simulink library "Delft_Tyre_dtlib"  (Simulink 6.4)
libraries: Delft_Tyre_sm1glib x2
settings Model: Creator=kozlowskimk  LastModifiedBy=hofstadrhmtvd

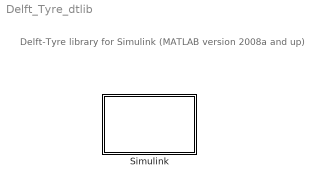
== system Delft_Tyre_dtlib ==
  note: Delft-Tyre library for Simulink
      | (MATLAB version 2008a and up)
  Simulink : Subsystem

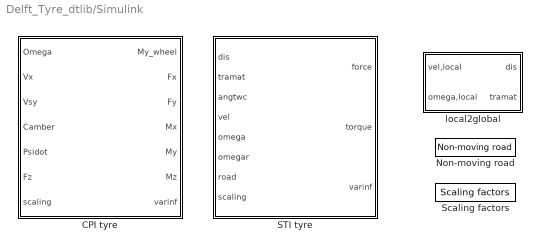
== system Delft_Tyre_dtlib/Simulink ==
  CPI tyre : Subsystem  Tag=CPI tyre  mask(CPI_tyre){idtyre=1, tpfname=, side_mode=(1xxx) left, dyn_mode=(xx0x) steady-state, mf_mode=(xxx0) none, use_mode=1e8, disp_debug=off}
      mask prompts: idtyre "Tyre ID [integer]"; tpfname "Tyre property file [string]"; side_mode "Tyre side            :"; dyn_mode "Dynamics           :"; mf_mode "Slip forces          :"; use_mode "Optional: use mode (overrides pop-up) [integer]"; disp_debug "Display debug messages"
      mask help:
      | Tyre model using the contact point interface (CPI). Inputs to the tyre model are the sliding velocities at the tyre-road contact point.
      |
      | Tyre model version: MF-Tyre/MF-Swift 6.2
      | © 1996-2013 TNO, Helmond, The Netherlands
      mask init:
      | if (abs(use_mode) > 4535 )
      |   iswtch=1000*side_mode+10*(dyn_mode-1)+(mf_mode-1);
      |   if (disp_debug) disp(['Delft-Tyre ' num2str(idtyre) ' -> use_mode=' num2str(iswtch) ]); end
      | else
      |   iswtch=use_mode;
      | end
      | 
      | 
      | if ~exist(tpfname)
      |     error('Tyre property file does not exist') 
      | end
      mask Help: eval('DTOpenHelp(504)')
      mask StyleString: edit,edit,popup((1xxx) left|(2xxx) right|(3xxx) symmetric),popup((xx0x) steady-state|(xx1x) relaxation behaviour|(xx2x) relaxation behaviour - non-linear),popup((xxx0) none|(xxx1) longitudinal|(xxx2) lateral|(xxx3) uncombined|(xxx4) combined|(xxx5) combined+turnslip),edit,checkbox
      mask CallbackString:
      | ||promtstr = get_param(gcb,'MaskPromptString');
      | index = find(double(promtstr)==124);
      | maskval = get_param(gcb,'MaskValues');
      | new_mode = [maskval{3}(2) '0' maskval{4}(4) maskval{5}(5)];
      | newpromtstr = [promtstr(1:index(5)) ['Optional: use mode (overrides pop-up) [current selection: ' new_mode ']'] promtstr(index(6):end)];
      | set_param(gcb,'MaskPromptString',newpromtstr);|promtstr = get_param(gcb,'MaskPromptString');
      | index = find(double(promtstr)==124);
      | maskval = get_param(gcb,'MaskValues');
      | new_mode = [maskval{3}(2) '0' maskval{4}(4) maskval{5}(5)];
      | newpromtstr = [promtstr(1:index(5)) ['Optional: use mode (overrides pop-up) [current selection: ' new_mode ']'] promtstr(index(6):end)];
      | set_param(gcb,'MaskPromptString',newpromtstr);|promtstr = get_param(gcb,'MaskPromptString');
      | index = find(double(promtstr)==124);
      | maskval = get_param(gcb,'MaskValues');
      | new_mode = [maskval{3}(2) '0' maskval{4}(4) maskval{5}(5)];
      | newpromtstr = [promtstr(1:index(5)) ['Optional: use mode (overrides pop-up) [current selection: ' new_mode ']'] promtstr(index(6):end)];
      | set_param(gcb,'MaskPromptString',newpromtstr);||
      mask Display:
      | text(0.3*160,0.7*178,'TNO Delft-Tyre')
      | plot(89.*[0.8828 0.8769 0.8597 0.7299 0.7043 0.6745 0.6443 0.6195 0.5884 0.5712 0.5653 0.5573 0.5346 0.4985 0.4515 0.3965 0.3373 ]+160/2-0.43*89,89.*[0.3654 0.3482 0.3335 0.2583 0.2486 0.2453 0.2486 0.2583 0.2764 0.2911 0.3083 0.2449 0.1945 0.1609 0.1462 0.1520 0.1768 ]+0.3*89)
      | plot(89.*[0.3255 0.3889 0.3965 0.4112 0.4313 0.3767 ]+160/2-0.43*89,89.*[0.1491 0.1222 0.1520 0.1777 0.1949 0.2184 ]+0.3*89)
      | plot(89.*[0.3553 0.4112 0.4633 0.4826 0.5464 ]+160/2-0.43*89,89.*[0.2012 0.1777 0.1722 0.1898 0.2268 ]+0.3*89)
      | plot(89.*[0.5426 0.5262 0.4826 0.4313 0.5603 0.5603 0.5065 ]+160/2-0.43*89,89.*[0.2184 0.2037 0.1898 0.1949 0.2692 0.2701 0.2932 ]+0.3*89)
      | plot(89.*[0.5279 0.5460 0.4868 ]+160/2-0.43*89,89.*[0.3007 0.2969 0.3402 ]+0.3*89)
      | plot(89.*[0.5279 0.5624 ]+160/2-0.43*89,89.*[0.3007 0.2856 ]+0.3*89)
      | plot(89.*[0.5628 0.5460 ]+160/2-0.43*89,89.*[0.2898 0.2969 ]+0.3*89)
      | plot(89.*[0.5712 0.5628 0.5573 ]+160/2-0.43*89,89.*[0.2911 0.2222 0.2449 ]+0.3*89)
      | plot(89.*[0.5586 0.5422 0.5082 0.4633 0.4515 0.4481 0.3889 0.3902 0.4544 0.5099 0.5523 0.5792 0.5884 ]+160/2-0.43*89,89.*[0.2541 0.2180 0.1861 0.1722 0.1462 0.1163 0.1222 0.0928 0.0865 0.1033 0.1428 0.2016 0.2764 ]+0.3*89)
      | plot(89.*[0.6195 0.6090 0.5792 0.5628 0.5380 0.5346 0.5422 ]+160/2-0.43*89,89.*[0.2583 0.1751 0.2016 0.2222 0.1680 0.1945 0.2180 ]+0.3*89)
      | plot(89.*[0.5262 0.5082 0.4985 0.4994 0.5380 0.5523 0.5792 0.6090 0.6333 0.6443 ]+160/2-0.43*89,89.*[0.2037 0.1861 0.1609 0.1319 0.1680 0.1428 0.1092 0.1751 0.1596 0.2486 ]+0.3*89)
      | plot(89.*[0.6745 0.6627 0.6333 0.6018 0.5792 0.5317 0.5099 0.4994 0.4481 0.4544 0.4700 0.5317 0.5510 0.6018 0.6291 0.6627 0.6926 0.7043 ]+160/2-0.43*89,89.*[0.2453 0.1508 0.1596 0.0890 0.1092 0.0655 0.1033 0.1319 0.1163 0.0865 0.0462 0.0655 0.0416 0.0890 0.0764 0.1508 0.1508 0.2486 ]+0.3*89)
      | plot(89.*[0.7299 0.7178 0.6926 0.6577 0.6291 0.5758 0.5510 0.4851 0.4700 0.3986 0.3213 0.2440 0.1718 0.1100 0.0626 ]+160/2-0.43*89,89.*[0.2583 0.1596 0.1508 0.0739 0.0764 0.0269 0.0416 0.0210 0.0462 0.0533 0.0861 0.1424 0.2184 0.3087 0.4074 ]+0.3*89)
      | plot(89.*[0.0487 0.0995 0.1100 0.1323 0.1516 0.1760 0.1399 ]+160/2-0.43*89,89.*[0.4082 0.3028 0.3087 0.3213 0.3326 0.3469 0.4221 ]+0.3*89)
      | plot(89.*[0.1126 0.1516 0.2024 0.2234 0.2474 0.2709 0.4011 0.4200 0.4322 0.3847 0.3486 0.3255 ]+160/2-0.43*89,89.*[0.4141 0.3326 0.2579 0.2776 0.2969 0.3121 0.3872 0.3965 0.3982 0.4670 0.5426 0.6191 ]+0.3*89)
      | plot(89.*[0.3486 0.3410 0.3755 0.3847 ]+160/2-0.43*89,89.*[0.5426 0.5330 0.4616 0.4670 ]+0.3*89)
      | plot(89.*[0.3755 0.3570 0.3234 ]+160/2-0.43*89,89.*[0.4616 0.4511 0.5212 ]+0.3*89)
      | plot(89.*[0.3570 0.2272 0.1936 ]+160/2-0.43*89,89.*[0.4511 0.3759 0.4460 ]+0.3*89)
      | plot(89.*[0.1684 0.2029 0.2272 0.2709 0.3217 0.4519 0.4721 0.4868 0.4322 ]+160/2-0.43*89,89.*[0.4334 0.3625 0.3759 0.3121 0.2583 0.3331 0.3415 0.3402 0.3982 ]+0.3*89)
      | plot(89.*[0.4200 0.3755 ]+160/2-0.43*89,89.*[0.3965 0.4616 ]+0.3*89)
      | plot(89.*[0.3570 0.4011 0.4519 0.5065 0.5279 0.4721 0.4200 ]+160/2-0.43*89,89.*[0.4511 0.3872 0.3331 0.2932 0.3007 0.3415 0.3965 ]+0.3*89)
      | plot(89.*[0.5065 0.3767 0.3217 0.2995 0.2474 0.2029 0.1760 0.2234 0.2785 0.2995 0.3553 0.3767 ]+160/2-0.43*89,89.*[0.2932 0.2184 0.2583 0.2419 0.2969 0.3625 0.3469 0.2776 0.2197 0.2419 0.2012 0.2184 ]+0.3*89)
      | plot(89.*[0.3553 0.3373 0.2785 0.2617 0.2024 0.1873 0.1323 0.0899 0.0630 0.0542 0.0231 0.0059 0.0000 0.0113 0.0168 0.0332 0.0630 0.0878 0.1172 0.1470 0.1722 0.3024 0.3192 0.3255 0.3179 0.3121 0.2948 0.1651 0.1394 0.1470 0.1172 0.0878 0.0630 0.0332 0.0168 0.0113 0.0000 ]+160/2-0.43*89,89.*[0.2012 0.1768 0.2197 0.1957 0.2579 0.2402 0.3213 0.4099 0.4994 0.5846 0.6027 0.6174 0.6346 0.5271 0.5157 0.5078 0.4994 0.4964 0.4990 0.5061 0.5174 0.5922 0.6056 0.6191 0.6917 0.6745 0.6598 0.5846 0.5745 0.6350 0.6350 0.6434 0.6594 0.6858 0.7064 0.7291 0.6346 ]+0.3*89)
      | plot(89.*[0.0059 0.0168 ]+160/2-0.43*89,89.*[0.6174 0.7064 ]+0.3*89)
      | plot(89.*[0.0113 0.0454 0.0529 0.0181 0.0113 ]+160/2-0.43*89,89.*[0.7291 0.8034 0.8270 0.7497 0.7291 ]+0.3*89)
      | plot(89.*[0.0168 0.0487 0.0454 ]+160/2-0.43*89,89.*[0.7064 0.7770 0.8034 ]+0.3*89)
      | plot(89.*[0.0487 0.0626 0.0899 0.0630 0.0542 0.0794 0.0878 0.1126 0.0899 ]+160/2-0.43*89,89.*[0.7770 0.7518 0.7182 0.6594 0.5846 0.5745 0.6434 0.6976 0.7182 ]+0.3*89)
      | plot(89.*[0.1126 0.1399 0.1684 0.1936 0.2570 ]+160/2-0.43*89,89.*[0.6976 0.6854 0.6829 0.6905 0.7274 ]+0.3*89)
      | plot(89.*[0.3011 0.1722 0.1936 ]+160/2-0.43*89,89.*[0.7182 0.6438 0.6905 ]+0.3*89)
      | plot(89.*[0.1684 0.1470 0.1722 0.1651 0.1722 0.1936 0.3234 0.3410 0.3192 0.3121 0.3163 ]+160/2-0.43*89,89.*[0.6829 0.6350 0.6438 0.5846 0.5174 0.4460 0.5212 0.5330 0.6056 0.6745 0.7119 ]+0.3*89)
      | plot(89.*[0.3200 0.3179 ]+160/2-0.43*89,89.*[0.7102 0.6917 ]+0.3*89)
      | plot(89.*[0.3020 0.2948 0.3024 0.3234 ]+160/2-0.43*89,89.*[0.7178 0.6598 0.5922 0.5212 ]+0.3*89)
      | plot(89.*[0.1470 0.1394 0.1096 0.1172 0.1399 0.1760 0.1516 0.1323 0.1100 0.0995 0.0987 0.1688 0.1806 0.1999 0.3297 0.2566 0.1264 0.0701 0.0529 0.1084 0.1264 0.1999 ]+160/2-0.43*89,89.*[0.5061 0.5745 0.5716 0.6350 0.6854 0.7190 0.7341 0.7577 0.7959 0.8240 0.8530 0.8748 0.9005 0.9185 0.9933 0.9706 0.8958 0.8438 0.8270 0.8782 0.8958 0.9185 ]+0.3*89)
      | plot(89.*[0.1806 0.1084 0.0987 0.0454 ]+160/2-0.43*89,89.*[0.9005 0.8782 0.8530 0.8034 ]+0.3*89)
      | plot(89.*[0.0487 0.0995 0.1655 0.1688 ]+160/2-0.43*89,89.*[0.7770 0.8240 0.8446 0.8748 ]+0.3*89)
      | plot(89.*[0.1655 0.1718 0.1873 0.2024 0.2234 0.2474 0.2029 0.1760 0.2234 ]+160/2-0.43*89,89.*[0.8446 0.8148 0.7745 0.7497 0.7333 0.7283 0.7144 0.7190 0.7333 ]+0.3*89)
      | plot(89.*[0.2272 0.2478 ]+160/2-0.43*89,89.*[0.7215 0.7278 ]+0.3*89)
      | plot(89.*[0.2272 0.2029 0.1684 ]+160/2-0.43*89,89.*[0.7215 0.7144 0.6829 ]+0.3*89)
      | plot(89.*[0.1936 0.2272 ]+160/2-0.43*89,89.*[0.6905 0.7215 ]+0.3*89)
      | plot(89.*[0.2024 0.1516 0.1126 ]+160/2-0.43*89,89.*[0.7497 0.7341 0.6976 ]+0.3*89)
      | plot(89.*[0.0899 0.1323 0.1873 0.2520 0.2440 0.2428 0.2499 0.2650 0.2852 0.4150 0.4372 0.3528 0.3297 0.4150 0.5065 0.5279 0.5460 0.4586 0.4372 0.5279 ]+160/2-0.43*89,89.*[0.7182 0.7577 0.7745 0.7686 0.8076 0.8370 0.8669 0.8925 0.9097 0.9849 0.9920 1.0000 0.9933 0.9849 0.9458 0.9534 0.9500 0.9870 0.9920 0.9534 ]+0.3*89)
      | plot(89.*[0.5065 0.3767 0.2852 0.1999 ]+160/2-0.43*89,89.*[0.9458 0.8711 0.9097 0.9185 ]+0.3*89)
      | plot(89.*[0.1806 0.2650 0.3553 0.3767 ]+160/2-0.43*89,89.*[0.9005 0.8925 0.8538 0.8711 ]+0.3*89)
      | plot(89.*[0.3553 0.3373 0.2499 0.1688 ]+160/2-0.43*89,89.*[0.8538 0.8295 0.8669 0.8748 ]+0.3*89)
      | plot(89.*[0.1655 0.2428 0.3255 0.3373 ]+160/2-0.43*89,89.*[0.8446 0.8370 0.8018 0.8295 ]+0.3*89)
      | plot(89.*[0.3255 0.3213 0.3213 0.3255 0.3373 0.2785 0.2617 0.3255 ]+160/2-0.43*89,89.*[0.8018 0.7749 0.7388 0.7165 0.7031 0.7278 0.7438 0.7165 ]+0.3*89)
      | plot(89.*[0.3213 0.2520 0.2617 0.2024 ]+160/2-0.43*89,89.*[0.7388 0.7686 0.7438 0.7497 ]+0.3*89)
      | plot(89.*[0.2234 0.2785 ]+160/2-0.43*89,89.*[0.7333 0.7278 ]+0.3*89)
      | plot(89.*[0.2869 0.2474 ]+160/2-0.43*89,89.*[0.7241 0.7283 ]+0.3*89)
      | plot(89.*[0.2440 0.3213 0.3986 0.4078 0.4246 0.4456 0.4683 0.5981 0.6182 0.6329 0.5460 ]+160/2-0.43*89,89.*[0.8076 0.7749 0.7186 0.7417 0.7661 0.7879 0.8043 0.8790 0.8874 0.8862 0.9500 ]+0.3*89)
      | plot(89.*[0.5279 0.6182 0.7022 0.7140 0.6329 ]+160/2-0.43*89,89.*[0.9534 0.8874 0.7984 0.8001 0.8862 ]+0.3*89)
      | plot(89.*[0.5981 0.5065 ]+160/2-0.43*89,89.*[0.8790 0.9458 ]+0.3*89)
      | plot(89.*[0.5981 0.6829 0.7022 ]+160/2-0.43*89,89.*[0.8790 0.7892 0.7984 ]+0.3*89)
      | plot(89.*[0.6829 0.5535 0.4683 0.3767 ]+160/2-0.43*89,89.*[0.7892 0.7144 0.8043 0.8711 ]+0.3*89)
      | plot(89.*[0.3553 0.4456 0.5300 0.5535 ]+160/2-0.43*89,89.*[0.8538 0.7879 0.6989 0.7144 ]+0.3*89)
      | plot(89.*[0.5300 0.5061 0.4246 0.3373 ]+160/2-0.43*89,89.*[0.6989 0.6800 0.7661 0.8295 ]+0.3*89)
      | plot(89.*[0.3255 0.4078 0.4851 0.5061 ]+160/2-0.43*89,89.*[0.8018 0.7417 0.6602 0.6800 ]+0.3*89)
      | plot(89.*[0.4851 0.4700 0.3986 0.3902 0.3889 0.4481 0.4544 0.4700 ]+160/2-0.43*89,89.*[0.6602 0.6426 0.7186 0.6884 0.6703 0.6077 0.6203 0.6426 ]+0.3*89)
      | plot(89.*[0.4851 0.5510 0.5758 0.6027 0.6262 0.7560 0.7745 0.7841 0.7140 ]+160/2-0.43*89,89.*[0.6602 0.5632 0.5779 0.5930 0.6069 0.6816 0.6926 0.6980 0.8001 ]+0.3*89)
      | plot(89.*[0.7022 0.7745 ]+160/2-0.43*89,89.*[0.7984 0.6926 ]+0.3*89)
      | plot(89.*[0.7841 0.8375 0.8303 0.7745 ]+160/2-0.43*89,89.*[0.6980 0.5863 0.5766 0.6926 ]+0.3*89)
      | plot(89.*[0.7560 0.6829 ]+160/2-0.43*89,89.*[0.6816 0.7892 ]+0.3*89)
      | plot(89.*[0.7560 0.8123 0.8303 ]+160/2-0.43*89,89.*[0.6816 0.5649 0.5766 ]+0.3*89)
      | plot(89.*[0.8123 0.6825 0.6262 0.5535 ]+160/2-0.43*89,89.*[0.5649 0.4901 0.6069 0.7144 ]+0.3*89)
      | plot(89.*[0.5300 0.6027 0.6577 0.6825 ]+160/2-0.43*89,89.*[0.6989 0.5930 0.4775 0.4901 ]+0.3*89)
      | plot(89.*[0.6577 0.6291 0.5758 0.5061 ]+160/2-0.43*89,89.*[0.4775 0.4658 0.5779 0.6800 ]+0.3*89)
      | plot(89.*[0.4700 0.5317 0.5510 0.6018 0.6291 ]+160/2-0.43*89,89.*[0.6426 0.5523 0.5632 0.4578 0.4658 ]+0.3*89)
      | plot(89.*[0.6018 0.5792 0.5317 0.5099 0.4544 0.3902 0.3213 ]+160/2-0.43*89,89.*[0.4578 0.4536 0.5523 0.5397 0.6203 0.6884 0.7388 ]+0.3*89)
      | plot(89.*[0.3255 0.3889 0.3965 0.4515 0.4481 0.4994 0.5099 0.5523 0.5792 ]+160/2-0.43*89,89.*[0.7165 0.6703 0.6602 0.6018 0.6077 0.5334 0.5397 0.4511 0.4536 ]+0.3*89)
      | plot(89.*[0.6018 0.6333 0.6627 0.6926 0.7178 0.8475 0.8652 0.8711 0.8375 ]+160/2-0.43*89,89.*[0.4578 0.3503 0.3524 0.3599 0.3713 0.4460 0.4595 0.4729 0.5863 ]+0.3*89)
      | plot(89.*[0.8303 0.8652 ]+160/2-0.43*89,89.*[0.5766 0.4595 ]+0.3*89)
      | plot(89.*[0.8711 0.8828 0.8711 0.8652 0.8475 0.7178 0.6825 0.6577 0.6027 0.5758 0.5061 0.4851 0.4078 0.3986 0.3902 0.3213 0.2520 0.1873 0.1718 0.1655 0.0995 0.0987 0.1688 0.1655 0.2428 0.2440 0.2520 0.2617 0.3255 0.3373 ]+160/2-0.43*89,89.*[0.4729 0.3654 0.2713 0.2503 0.2348 0.1596 0.0815 0.0739 0.0223 0.0269 0.0050 0.0210 0.0290 0.0533 0.0928 0.1222 0.1726 0.2402 0.2184 0.2058 0.3028 0.3020 0.1999 0.2058 0.1243 0.1424 0.1726 0.1957 0.1491 0.1768 ]+0.3*89)
      | plot(89.*[0.3255 0.3213 0.3213 0.3255 0.4078 0.4246 0.5061 0.5300 0.6027 0.6262 0.6825 0.8123 0.8475 0.8597 0.8475 0.8123 ]+160/2-0.43*89,89.*[0.1491 0.1222 0.0861 0.0643 0.0290 0.0130 0.0050 0.0000 0.0223 0.0294 0.0815 0.1562 0.2348 0.3335 0.4460 0.5649 ]+0.3*89)
      | plot(89.*[0.8652 0.8769 0.8652 0.8303 0.8123 0.7560 0.6262 0.5535 0.5300 0.4456 0.4246 0.3373 0.3255 0.2428 0.2499 0.3373 ]+160/2-0.43*89,89.*[0.4595 0.3482 0.2503 0.1735 0.1562 0.1046 0.0294 0.0067 0.0000 0.0084 0.0130 0.0504 0.0643 0.1243 0.1138 0.0504 ]+0.3*89)
      | plot(89.*[0.0487 0.0168 0.0059 ]+160/2-0.43*89,89.*[0.4082 0.5157 0.6174 ]+0.3*89)
      | plot(89.*[0.0231 0.0332 0.0626 0.1100 0.1718 0.2440 ]+160/2-0.43*89,89.*[0.6027 0.6858 0.7518 0.7959 0.8148 0.8076 ]+0.3*89)
      | plot(89.*[0.3373 0.3965 ]+160/2-0.43*89,89.*[0.7031 0.6602 ]+0.3*89)
      | plot(89.*[0.4515 0.4985 0.4994 0.5380 0.5523 0.5792 0.6090 0.6333 0.6443 ]+160/2-0.43*89,89.*[0.6018 0.5330 0.5334 0.4519 0.4511 0.3612 0.3532 0.3503 0.2486 ]+0.3*89)
      | plot(89.*[0.6745 0.6627 0.6291 ]+160/2-0.43*89,89.*[0.2453 0.3524 0.4658 ]+0.3*89)
      | plot(89.*[0.6577 0.6926 0.7043 ]+160/2-0.43*89,89.*[0.4775 0.3599 0.2486 ]+0.3*89)
      | plot(89.*[0.7299 0.7178 0.6825 ]+160/2-0.43*89,89.*[0.2583 0.3713 0.4901 ]+0.3*89)
      | plot(89.*[0.5792 0.6090 0.6195 ]+160/2-0.43*89,89.*[0.4536 0.3532 0.2583 ]+0.3*89)
      | plot(89.*[0.5884 0.5792 0.5628 0.5380 0.5346 0.5573 0.5628 0.5712 ]+160/2-0.43*89,89.*[0.2764 0.3612 0.3692 0.4519 0.4578 0.3809 0.3692 0.2911 ]+0.3*89)
      | plot(89.*[0.5653 0.5573 ]+160/2-0.43*89,89.*[0.3083 0.3809 ]+0.3*89)
      | plot(89.*[0.5346 0.4985 ]+160/2-0.43*89,89.*[0.4578 0.5330 ]+0.3*89)
      | plot(89.*[0.1470 0.1684 0.1936 ]+160/2-0.43*89,89.*[0.5061 0.4334 0.4460 ]+0.3*89)
      | plot(89.*[0.1684 0.1399 0.1172 0.1096 0.0794 0.0878 0.1126 0.1399 ]+160/2-0.43*89,89.*[0.4334 0.4221 0.4990 0.5716 0.5745 0.4964 0.4141 0.4221 ]+0.3*89)
      | plot(89.*[0.1126 0.0899 0.0626 0.0332 0.0231 ]+160/2-0.43*89,89.*[0.4141 0.4099 0.4074 0.5078 0.6027 ]+0.3*89)
      | plot(89.*[0.0113 0.0454 0.0487 0.0626 ]+160/2-0.43*89,89.*[0.5271 0.4137 0.4082 0.4074 ]+0.3*89)
      | plot(89.*[0.0454 0.0987 ]+160/2-0.43*89,89.*[0.4137 0.3020 ]+0.3*89)
  Non-moving road : Delft_Tyre_sm1glib/SimMechanics 1G/Non-moving road  Tag=Non-moving road  SystemSampleTime=-1  dummy=off
  STI tyre : Subsystem  Tag=STI tyre  mask(STI_tyre){idtyre=1, tpfname=, rdfname='', side_mode=(1xxx) left, cnt_mode=(x1xx) smooth road, dyn_mode=(xx0x) steady-state, mf_mode=(xxx0) none, use_mode=1e8, disp_debug=off}
      mask prompts: idtyre "Tyre ID [integer]"; tpfname "Tyre properties [string or struct]"; rdfname "Road data file (may be empty) [string]"; side_mode "Tyre side            :"; cnt_mode "Contact method :"; dyn_mode "Dynamics           :"; mf_mode "Slip forces          :"; use_mode "Optional: use mode (overrides pop-up) [integer]"; disp_debug "Display debug messages"
      mask help:
      | Tyre model using the standard tyre interface (STI), as developed by the TYDEX workgroup. Inputs to the tyre model are the motions at the wheel centre. The outputs force and torque should also be applied to the wheel centre.
      |
      | Tyre model version: MF-Tyre/MF-Swift 6.2
      | © 1996-2013 TNO, Helmond, The Netherlands
      mask init:
      | idroad=1;
      | if (abs(use_mode) > 4535 )
      |   iswtch=1000*side_mode+100*cnt_mode+10*(dyn_mode-1)+(mf_mode-1);
      |   if (disp_debug) disp(['Delft-Tyre ' num2str(idtyre) ' -> use_mode=' num2str(iswtch) ]); end
      | else
      |   iswtch=use_mode;
      | end
      | 
      | % switch between tpf file or struct
      | if ischar(tpfname)
      |     typarr=zeros(300,1);
      |     tpfname_dummy=tpfname;
      | elseif isstruct(tpfname)
      |     typarr=tno_tpf_struct2array(tpfname,idtyre);
      |     tpfname_dummy='';
      | else
      |     typarr=zeros(300,1);
      |     tpfname_dummy='';
      |     error(['Mask parameter ''Tyre property file'' should be supplied as string or structure for tyre ' num2str(idtyre)])
      | end
      mask Help: eval('DTOpenHelp(505)')
      mask StyleString: edit,edit,edit,popup((1xxx) left|(2xxx) right|(3xxx) symmetric),popup((x1xx) smooth road|(x2xx) smooth road (motorcycle: circular cross section)|(x3xx) moving road|(x4xx) 2D short wavelength road contact|(x5xx) 3D short wavelength road contact),popup((xx0x) steady-state|(xx1x) relaxation behaviour|(xx2x) relaxation behaviour - non-linear|(xx3x) rigid ring|(xx4x) rigid ring + initial statics),popup((xxx0) none|(xxx1) longitudinal|(xxx2) lateral|(xxx3) uncombined|(xxx4) combined|(xxx5) combined+turnslip),edit,checkbox
      mask CallbackString:
      | |||promtstr = get_param(gcb,'MaskPromptString');
      | index = find(double(promtstr)==124);
      | maskval = get_param(gcb,'MaskValues');
      | new_mode = [maskval{4}(2) maskval{5}(3) maskval{6}(4) maskval{7}(5)];
      | newpromtstr = [promtstr(1:index(7)) ['Optional: use mode (overrides pop-up) [current selection: ' new_mode ']'] promtstr(index(8):end)];
      | set_param(gcb,'MaskPromptString',newpromtstr);|promtstr = get_param(gcb,'MaskPromptString');
      | index = find(double(promtstr)==124);
      | maskval = get_param(gcb,'MaskValues');
      | new_mode = [maskval{4}(2) maskval{5}(3) maskval{6}(4) maskval{7}(5)];
      | newpromtstr = [promtstr(1:index(7)) ['Optional: use mode (overrides pop-up) [current selection: ' new_mode ']'] promtstr(index(8):end)];
      | set_param(gcb,'MaskPromptString',newpromtstr);|promtstr = get_param(gcb,'MaskPromptString');
      | index = find(double(promtstr)==124);
      | maskval = get_param(gcb,'MaskValues');
      | new_mode = [maskval{4}(2) maskval{5}(3) maskval{6}(4) maskval{7}(5)];
      | newpromtstr = [promtstr(1:index(7)) ['Optional: use mode (overrides pop-up) [current selection: ' new_mode ']'] promtstr(index(8):end)];
      | set_param(gcb,'MaskPromptString',newpromtstr);|promtstr = get_param(gcb,'MaskPromptString');
      | index = find(double(promtstr)==124);
      | maskval = get_param(gcb,'MaskValues');
      | new_mode = [maskval{4}(2) maskval{5}(3) maskval{6}(4) maskval{7}(5)];
      | newpromtstr = [promtstr(1:index(7)) ['Optional: use mode (overrides pop-up) [current selection: ' new_mode ']'] promtstr(index(8):end)];
      | set_param(gcb,'MaskPromptString',newpromtstr);||
      mask Display:
      | text(0.3*160,0.7*178,'TNO Delft-Tyre')
      | plot(89.*[0.8828 0.8769 0.8597 0.7299 0.7043 0.6745 0.6443 0.6195 0.5884 0.5712 0.5653 0.5573 0.5346 0.4985 0.4515 0.3965 0.3373 ]+160/2-0.43*89,89.*[0.3654 0.3482 0.3335 0.2583 0.2486 0.2453 0.2486 0.2583 0.2764 0.2911 0.3083 0.2449 0.1945 0.1609 0.1462 0.1520 0.1768 ]+0.3*89)
      | plot(89.*[0.3255 0.3889 0.3965 0.4112 0.4313 0.3767 ]+160/2-0.43*89,89.*[0.1491 0.1222 0.1520 0.1777 0.1949 0.2184 ]+0.3*89)
      | plot(89.*[0.3553 0.4112 0.4633 0.4826 0.5464 ]+160/2-0.43*89,89.*[0.2012 0.1777 0.1722 0.1898 0.2268 ]+0.3*89)
      | plot(89.*[0.5426 0.5262 0.4826 0.4313 0.5603 0.5603 0.5065 ]+160/2-0.43*89,89.*[0.2184 0.2037 0.1898 0.1949 0.2692 0.2701 0.2932 ]+0.3*89)
      | plot(89.*[0.5279 0.5460 0.4868 ]+160/2-0.43*89,89.*[0.3007 0.2969 0.3402 ]+0.3*89)
      | plot(89.*[0.5279 0.5624 ]+160/2-0.43*89,89.*[0.3007 0.2856 ]+0.3*89)
      | plot(89.*[0.5628 0.5460 ]+160/2-0.43*89,89.*[0.2898 0.2969 ]+0.3*89)
      | plot(89.*[0.5712 0.5628 0.5573 ]+160/2-0.43*89,89.*[0.2911 0.2222 0.2449 ]+0.3*89)
      | plot(89.*[0.5586 0.5422 0.5082 0.4633 0.4515 0.4481 0.3889 0.3902 0.4544 0.5099 0.5523 0.5792 0.5884 ]+160/2-0.43*89,89.*[0.2541 0.2180 0.1861 0.1722 0.1462 0.1163 0.1222 0.0928 0.0865 0.1033 0.1428 0.2016 0.2764 ]+0.3*89)
      | plot(89.*[0.6195 0.6090 0.5792 0.5628 0.5380 0.5346 0.5422 ]+160/2-0.43*89,89.*[0.2583 0.1751 0.2016 0.2222 0.1680 0.1945 0.2180 ]+0.3*89)
      | plot(89.*[0.5262 0.5082 0.4985 0.4994 0.5380 0.5523 0.5792 0.6090 0.6333 0.6443 ]+160/2-0.43*89,89.*[0.2037 0.1861 0.1609 0.1319 0.1680 0.1428 0.1092 0.1751 0.1596 0.2486 ]+0.3*89)
      | plot(89.*[0.6745 0.6627 0.6333 0.6018 0.5792 0.5317 0.5099 0.4994 0.4481 0.4544 0.4700 0.5317 0.5510 0.6018 0.6291 0.6627 0.6926 0.7043 ]+160/2-0.43*89,89.*[0.2453 0.1508 0.1596 0.0890 0.1092 0.0655 0.1033 0.1319 0.1163 0.0865 0.0462 0.0655 0.0416 0.0890 0.0764 0.1508 0.1508 0.2486 ]+0.3*89)
      | plot(89.*[0.7299 0.7178 0.6926 0.6577 0.6291 0.5758 0.5510 0.4851 0.4700 0.3986 0.3213 0.2440 0.1718 0.1100 0.0626 ]+160/2-0.43*89,89.*[0.2583 0.1596 0.1508 0.0739 0.0764 0.0269 0.0416 0.0210 0.0462 0.0533 0.0861 0.1424 0.2184 0.3087 0.4074 ]+0.3*89)
      | plot(89.*[0.0487 0.0995 0.1100 0.1323 0.1516 0.1760 0.1399 ]+160/2-0.43*89,89.*[0.4082 0.3028 0.3087 0.3213 0.3326 0.3469 0.4221 ]+0.3*89)
      | plot(89.*[0.1126 0.1516 0.2024 0.2234 0.2474 0.2709 0.4011 0.4200 0.4322 0.3847 0.3486 0.3255 ]+160/2-0.43*89,89.*[0.4141 0.3326 0.2579 0.2776 0.2969 0.3121 0.3872 0.3965 0.3982 0.4670 0.5426 0.6191 ]+0.3*89)
      | plot(89.*[0.3486 0.3410 0.3755 0.3847 ]+160/2-0.43*89,89.*[0.5426 0.5330 0.4616 0.4670 ]+0.3*89)
      | plot(89.*[0.3755 0.3570 0.3234 ]+160/2-0.43*89,89.*[0.4616 0.4511 0.5212 ]+0.3*89)
      | plot(89.*[0.3570 0.2272 0.1936 ]+160/2-0.43*89,89.*[0.4511 0.3759 0.4460 ]+0.3*89)
      | plot(89.*[0.1684 0.2029 0.2272 0.2709 0.3217 0.4519 0.4721 0.4868 0.4322 ]+160/2-0.43*89,89.*[0.4334 0.3625 0.3759 0.3121 0.2583 0.3331 0.3415 0.3402 0.3982 ]+0.3*89)
      | plot(89.*[0.4200 0.3755 ]+160/2-0.43*89,89.*[0.3965 0.4616 ]+0.3*89)
      | plot(89.*[0.3570 0.4011 0.4519 0.5065 0.5279 0.4721 0.4200 ]+160/2-0.43*89,89.*[0.4511 0.3872 0.3331 0.2932 0.3007 0.3415 0.3965 ]+0.3*89)
      | plot(89.*[0.5065 0.3767 0.3217 0.2995 0.2474 0.2029 0.1760 0.2234 0.2785 0.2995 0.3553 0.3767 ]+160/2-0.43*89,89.*[0.2932 0.2184 0.2583 0.2419 0.2969 0.3625 0.3469 0.2776 0.2197 0.2419 0.2012 0.2184 ]+0.3*89)
      | plot(89.*[0.3553 0.3373 0.2785 0.2617 0.2024 0.1873 0.1323 0.0899 0.0630 0.0542 0.0231 0.0059 0.0000 0.0113 0.0168 0.0332 0.0630 0.0878 0.1172 0.1470 0.1722 0.3024 0.3192 0.3255 0.3179 0.3121 0.2948 0.1651 0.1394 0.1470 0.1172 0.0878 0.0630 0.0332 0.0168 0.0113 0.0000 ]+160/2-0.43*89,89.*[0.2012 0.1768 0.2197 0.1957 0.2579 0.2402 0.3213 0.4099 0.4994 0.5846 0.6027 0.6174 0.6346 0.5271 0.5157 0.5078 0.4994 0.4964 0.4990 0.5061 0.5174 0.5922 0.6056 0.6191 0.6917 0.6745 0.6598 0.5846 0.5745 0.6350 0.6350 0.6434 0.6594 0.6858 0.7064 0.7291 0.6346 ]+0.3*89)
      | plot(89.*[0.0059 0.0168 ]+160/2-0.43*89,89.*[0.6174 0.7064 ]+0.3*89)
      | plot(89.*[0.0113 0.0454 0.0529 0.0181 0.0113 ]+160/2-0.43*89,89.*[0.7291 0.8034 0.8270 0.7497 0.7291 ]+0.3*89)
      | plot(89.*[0.0168 0.0487 0.0454 ]+160/2-0.43*89,89.*[0.7064 0.7770 0.8034 ]+0.3*89)
      | plot(89.*[0.0487 0.0626 0.0899 0.0630 0.0542 0.0794 0.0878 0.1126 0.0899 ]+160/2-0.43*89,89.*[0.7770 0.7518 0.7182 0.6594 0.5846 0.5745 0.6434 0.6976 0.7182 ]+0.3*89)
      | plot(89.*[0.1126 0.1399 0.1684 0.1936 0.2570 ]+160/2-0.43*89,89.*[0.6976 0.6854 0.6829 0.6905 0.7274 ]+0.3*89)
      | plot(89.*[0.3011 0.1722 0.1936 ]+160/2-0.43*89,89.*[0.7182 0.6438 0.6905 ]+0.3*89)
      | plot(89.*[0.1684 0.1470 0.1722 0.1651 0.1722 0.1936 0.3234 0.3410 0.3192 0.3121 0.3163 ]+160/2-0.43*89,89.*[0.6829 0.6350 0.6438 0.5846 0.5174 0.4460 0.5212 0.5330 0.6056 0.6745 0.7119 ]+0.3*89)
      | plot(89.*[0.3200 0.3179 ]+160/2-0.43*89,89.*[0.7102 0.6917 ]+0.3*89)
      | plot(89.*[0.3020 0.2948 0.3024 0.3234 ]+160/2-0.43*89,89.*[0.7178 0.6598 0.5922 0.5212 ]+0.3*89)
      | plot(89.*[0.1470 0.1394 0.1096 0.1172 0.1399 0.1760 0.1516 0.1323 0.1100 0.0995 0.0987 0.1688 0.1806 0.1999 0.3297 0.2566 0.1264 0.0701 0.0529 0.1084 0.1264 0.1999 ]+160/2-0.43*89,89.*[0.5061 0.5745 0.5716 0.6350 0.6854 0.7190 0.7341 0.7577 0.7959 0.8240 0.8530 0.8748 0.9005 0.9185 0.9933 0.9706 0.8958 0.8438 0.8270 0.8782 0.8958 0.9185 ]+0.3*89)
      | plot(89.*[0.1806 0.1084 0.0987 0.0454 ]+160/2-0.43*89,89.*[0.9005 0.8782 0.8530 0.8034 ]+0.3*89)
      | plot(89.*[0.0487 0.0995 0.1655 0.1688 ]+160/2-0.43*89,89.*[0.7770 0.8240 0.8446 0.8748 ]+0.3*89)
      | plot(89.*[0.1655 0.1718 0.1873 0.2024 0.2234 0.2474 0.2029 0.1760 0.2234 ]+160/2-0.43*89,89.*[0.8446 0.8148 0.7745 0.7497 0.7333 0.7283 0.7144 0.7190 0.7333 ]+0.3*89)
      | plot(89.*[0.2272 0.2478 ]+160/2-0.43*89,89.*[0.7215 0.7278 ]+0.3*89)
      | plot(89.*[0.2272 0.2029 0.1684 ]+160/2-0.43*89,89.*[0.7215 0.7144 0.6829 ]+0.3*89)
      | plot(89.*[0.1936 0.2272 ]+160/2-0.43*89,89.*[0.6905 0.7215 ]+0.3*89)
      | plot(89.*[0.2024 0.1516 0.1126 ]+160/2-0.43*89,89.*[0.7497 0.7341 0.6976 ]+0.3*89)
      | plot(89.*[0.0899 0.1323 0.1873 0.2520 0.2440 0.2428 0.2499 0.2650 0.2852 0.4150 0.4372 0.3528 0.3297 0.4150 0.5065 0.5279 0.5460 0.4586 0.4372 0.5279 ]+160/2-0.43*89,89.*[0.7182 0.7577 0.7745 0.7686 0.8076 0.8370 0.8669 0.8925 0.9097 0.9849 0.9920 1.0000 0.9933 0.9849 0.9458 0.9534 0.9500 0.9870 0.9920 0.9534 ]+0.3*89)
      | plot(89.*[0.5065 0.3767 0.2852 0.1999 ]+160/2-0.43*89,89.*[0.9458 0.8711 0.9097 0.9185 ]+0.3*89)
      | plot(89.*[0.1806 0.2650 0.3553 0.3767 ]+160/2-0.43*89,89.*[0.9005 0.8925 0.8538 0.8711 ]+0.3*89)
      | plot(89.*[0.3553 0.3373 0.2499 0.1688 ]+160/2-0.43*89,89.*[0.8538 0.8295 0.8669 0.8748 ]+0.3*89)
      | plot(89.*[0.1655 0.2428 0.3255 0.3373 ]+160/2-0.43*89,89.*[0.8446 0.8370 0.8018 0.8295 ]+0.3*89)
      | plot(89.*[0.3255 0.3213 0.3213 0.3255 0.3373 0.2785 0.2617 0.3255 ]+160/2-0.43*89,89.*[0.8018 0.7749 0.7388 0.7165 0.7031 0.7278 0.7438 0.7165 ]+0.3*89)
      | plot(89.*[0.3213 0.2520 0.2617 0.2024 ]+160/2-0.43*89,89.*[0.7388 0.7686 0.7438 0.7497 ]+0.3*89)
      | plot(89.*[0.2234 0.2785 ]+160/2-0.43*89,89.*[0.7333 0.7278 ]+0.3*89)
      | plot(89.*[0.2869 0.2474 ]+160/2-0.43*89,89.*[0.7241 0.7283 ]+0.3*89)
      | plot(89.*[0.2440 0.3213 0.3986 0.4078 0.4246 0.4456 0.4683 0.5981 0.6182 0.6329 0.5460 ]+160/2-0.43*89,89.*[0.8076 0.7749 0.7186 0.7417 0.7661 0.7879 0.8043 0.8790 0.8874 0.8862 0.9500 ]+0.3*89)
      | plot(89.*[0.5279 0.6182 0.7022 0.7140 0.6329 ]+160/2-0.43*89,89.*[0.9534 0.8874 0.7984 0.8001 0.8862 ]+0.3*89)
      | plot(89.*[0.5981 0.5065 ]+160/2-0.43*89,89.*[0.8790 0.9458 ]+0.3*89)
      | plot(89.*[0.5981 0.6829 0.7022 ]+160/2-0.43*89,89.*[0.8790 0.7892 0.7984 ]+0.3*89)
      | plot(89.*[0.6829 0.5535 0.4683 0.3767 ]+160/2-0.43*89,89.*[0.7892 0.7144 0.8043 0.8711 ]+0.3*89)
      | plot(89.*[0.3553 0.4456 0.5300 0.5535 ]+160/2-0.43*89,89.*[0.8538 0.7879 0.6989 0.7144 ]+0.3*89)
      | plot(89.*[0.5300 0.5061 0.4246 0.3373 ]+160/2-0.43*89,89.*[0.6989 0.6800 0.7661 0.8295 ]+0.3*89)
      | plot(89.*[0.3255 0.4078 0.4851 0.5061 ]+160/2-0.43*89,89.*[0.8018 0.7417 0.6602 0.6800 ]+0.3*89)
      | plot(89.*[0.4851 0.4700 0.3986 0.3902 0.3889 0.4481 0.4544 0.4700 ]+160/2-0.43*89,89.*[0.6602 0.6426 0.7186 0.6884 0.6703 0.6077 0.6203 0.6426 ]+0.3*89)
      | plot(89.*[0.4851 0.5510 0.5758 0.6027 0.6262 0.7560 0.7745 0.7841 0.7140 ]+160/2-0.43*89,89.*[0.6602 0.5632 0.5779 0.5930 0.6069 0.6816 0.6926 0.6980 0.8001 ]+0.3*89)
      | plot(89.*[0.7022 0.7745 ]+160/2-0.43*89,89.*[0.7984 0.6926 ]+0.3*89)
      | plot(89.*[0.7841 0.8375 0.8303 0.7745 ]+160/2-0.43*89,89.*[0.6980 0.5863 0.5766 0.6926 ]+0.3*89)
      | plot(89.*[0.7560 0.6829 ]+160/2-0.43*89,89.*[0.6816 0.7892 ]+0.3*89)
      | plot(89.*[0.7560 0.8123 0.8303 ]+160/2-0.43*89,89.*[0.6816 0.5649 0.5766 ]+0.3*89)
      | plot(89.*[0.8123 0.6825 0.6262 0.5535 ]+160/2-0.43*89,89.*[0.5649 0.4901 0.6069 0.7144 ]+0.3*89)
      | plot(89.*[0.5300 0.6027 0.6577 0.6825 ]+160/2-0.43*89,89.*[0.6989 0.5930 0.4775 0.4901 ]+0.3*89)
      | plot(89.*[0.6577 0.6291 0.5758 0.5061 ]+160/2-0.43*89,89.*[0.4775 0.4658 0.5779 0.6800 ]+0.3*89)
      | plot(89.*[0.4700 0.5317 0.5510 0.6018 0.6291 ]+160/2-0.43*89,89.*[0.6426 0.5523 0.5632 0.4578 0.4658 ]+0.3*89)
      | plot(89.*[0.6018 0.5792 0.5317 0.5099 0.4544 0.3902 0.3213 ]+160/2-0.43*89,89.*[0.4578 0.4536 0.5523 0.5397 0.6203 0.6884 0.7388 ]+0.3*89)
      | plot(89.*[0.3255 0.3889 0.3965 0.4515 0.4481 0.4994 0.5099 0.5523 0.5792 ]+160/2-0.43*89,89.*[0.7165 0.6703 0.6602 0.6018 0.6077 0.5334 0.5397 0.4511 0.4536 ]+0.3*89)
      | plot(89.*[0.6018 0.6333 0.6627 0.6926 0.7178 0.8475 0.8652 0.8711 0.8375 ]+160/2-0.43*89,89.*[0.4578 0.3503 0.3524 0.3599 0.3713 0.4460 0.4595 0.4729 0.5863 ]+0.3*89)
      | plot(89.*[0.8303 0.8652 ]+160/2-0.43*89,89.*[0.5766 0.4595 ]+0.3*89)
      | plot(89.*[0.8711 0.8828 0.8711 0.8652 0.8475 0.7178 0.6825 0.6577 0.6027 0.5758 0.5061 0.4851 0.4078 0.3986 0.3902 0.3213 0.2520 0.1873 0.1718 0.1655 0.0995 0.0987 0.1688 0.1655 0.2428 0.2440 0.2520 0.2617 0.3255 0.3373 ]+160/2-0.43*89,89.*[0.4729 0.3654 0.2713 0.2503 0.2348 0.1596 0.0815 0.0739 0.0223 0.0269 0.0050 0.0210 0.0290 0.0533 0.0928 0.1222 0.1726 0.2402 0.2184 0.2058 0.3028 0.3020 0.1999 0.2058 0.1243 0.1424 0.1726 0.1957 0.1491 0.1768 ]+0.3*89)
      | plot(89.*[0.3255 0.3213 0.3213 0.3255 0.4078 0.4246 0.5061 0.5300 0.6027 0.6262 0.6825 0.8123 0.8475 0.8597 0.8475 0.8123 ]+160/2-0.43*89,89.*[0.1491 0.1222 0.0861 0.0643 0.0290 0.0130 0.0050 0.0000 0.0223 0.0294 0.0815 0.1562 0.2348 0.3335 0.4460 0.5649 ]+0.3*89)
      | plot(89.*[0.8652 0.8769 0.8652 0.8303 0.8123 0.7560 0.6262 0.5535 0.5300 0.4456 0.4246 0.3373 0.3255 0.2428 0.2499 0.3373 ]+160/2-0.43*89,89.*[0.4595 0.3482 0.2503 0.1735 0.1562 0.1046 0.0294 0.0067 0.0000 0.0084 0.0130 0.0504 0.0643 0.1243 0.1138 0.0504 ]+0.3*89)
      | plot(89.*[0.0487 0.0168 0.0059 ]+160/2-0.43*89,89.*[0.4082 0.5157 0.6174 ]+0.3*89)
      | plot(89.*[0.0231 0.0332 0.0626 0.1100 0.1718 0.2440 ]+160/2-0.43*89,89.*[0.6027 0.6858 0.7518 0.7959 0.8148 0.8076 ]+0.3*89)
      | plot(89.*[0.3373 0.3965 ]+160/2-0.43*89,89.*[0.7031 0.6602 ]+0.3*89)
      | plot(89.*[0.4515 0.4985 0.4994 0.5380 0.5523 0.5792 0.6090 0.6333 0.6443 ]+160/2-0.43*89,89.*[0.6018 0.5330 0.5334 0.4519 0.4511 0.3612 0.3532 0.3503 0.2486 ]+0.3*89)
      | plot(89.*[0.6745 0.6627 0.6291 ]+160/2-0.43*89,89.*[0.2453 0.3524 0.4658 ]+0.3*89)
      | plot(89.*[0.6577 0.6926 0.7043 ]+160/2-0.43*89,89.*[0.4775 0.3599 0.2486 ]+0.3*89)
      | plot(89.*[0.7299 0.7178 0.6825 ]+160/2-0.43*89,89.*[0.2583 0.3713 0.4901 ]+0.3*89)
      | plot(89.*[0.5792 0.6090 0.6195 ]+160/2-0.43*89,89.*[0.4536 0.3532 0.2583 ]+0.3*89)
      | plot(89.*[0.5884 0.5792 0.5628 0.5380 0.5346 0.5573 0.5628 0.5712 ]+160/2-0.43*89,89.*[0.2764 0.3612 0.3692 0.4519 0.4578 0.3809 0.3692 0.2911 ]+0.3*89)
      | plot(89.*[0.5653 0.5573 ]+160/2-0.43*89,89.*[0.3083 0.3809 ]+0.3*89)
      | plot(89.*[0.5346 0.4985 ]+160/2-0.43*89,89.*[0.4578 0.5330 ]+0.3*89)
      | plot(89.*[0.1470 0.1684 0.1936 ]+160/2-0.43*89,89.*[0.5061 0.4334 0.4460 ]+0.3*89)
      | plot(89.*[0.1684 0.1399 0.1172 0.1096 0.0794 0.0878 0.1126 0.1399 ]+160/2-0.43*89,89.*[0.4334 0.4221 0.4990 0.5716 0.5745 0.4964 0.4141 0.4221 ]+0.3*89)
      | plot(89.*[0.1126 0.0899 0.0626 0.0332 0.0231 ]+160/2-0.43*89,89.*[0.4141 0.4099 0.4074 0.5078 0.6027 ]+0.3*89)
      | plot(89.*[0.0113 0.0454 0.0487 0.0626 ]+160/2-0.43*89,89.*[0.5271 0.4137 0.4082 0.4074 ]+0.3*89)
      | plot(89.*[0.0454 0.0987 ]+160/2-0.43*89,89.*[0.4137 0.3020 ]+0.3*89)
  Scaling factors : Delft_Tyre_sm1glib/SimMechanics 1G/Scaling factors  Tag=Scaling factors  SystemSampleTime=-1  LMUX=1  LKX=1  LMUY=1  LKY=1  LKYC=1  LTR=1  LKZC=1
  local2global : Subsystem  Tag=local2global  mask(local2global){init_pos=[0 0 0.29], init_angle=[0 0 0]}
      mask prompts: init_pos "Wheel center position (global)"; init_angle "Wheel center orientation (global, Bryant angles, rotation seq. ZXY). Angle input order [X Y Z]."
      mask help:
      | Transformation block to transform local (angular) velocities into a global position and orientation.
      | © 1996-2013 TNO, Helmond, The Netherlands
      mask Help:
      | <!doctype html public "-//w3c//dtd html 4.0 transitional//en">
      | <html>
      | <head>
      |    <meta http-equiv="Content-Type" content="text/html; charset=iso-8859-1">
      |    <meta name="GENERATOR" content="Mozilla/4.72 [en] (X11; I; SunOS 5.7 sun4u) [Netscape]">
      | </head>
      | <body>
      | <font size=+1><b>Position and orientation</b>: </font><font size="4">Calculation
      | of transformation matrix and global position from local HUB velocities</font>
      | <p><font size="4">Transforms the local translational and angular velocity of
      | the wheel center to the global position and transformation matrix for use with
      | the Standard
      | Tyre Interface (STI)</font></p>
      | <p>This block is supplied as addition for the possible
      | conversion needed to run localized input with MF-Tyre and SWIFT-Tyre implementing
      | the Standard Tyre Interface.<br>
      | <hr WIDTH="100%">
      | <br><font size=+1>Inputs:</font>
      | <ul>
      | <li>
      | <b>vel, &nbsp;local(3)</b>: local velocity of the wheel center expressed in the carrier
      | frame: x, y and z component</li>
      | 
      | <li>
      | <b>omega, local (3)</b>: local  angular velocity of the wheel carrier expressed
      | in the carrier frame: x, y and z component</li>
      | 
      | </ul>
      | 
      | <hr WIDTH="100%">
      | <br><font size=+1>Outputs:</font>
      | <ul>
      | <li>
      | <b>dis(3)</b>: location of the wheel center in the global frame: x, y and z
      | coordinate</li>
      | 
      |     <li><b>tramat(9)</b>: transformation matrix from wheel carrier to the global frame
      | <BR>tramat(1..3): representation of the unit x-vector of the carrier axis in the
      | global frame <BR>tramat(4..6): representation of the unit y-vector of the
      | carrier axis in the global frame <BR>tramat(7..9): representation of the unit
      | z-vector of the carrier axis in the global frame </li>
      | </ul>
      | 
      | <hr WIDTH="100%">
      | <br><font size=+1>Parameters:</font>
      | <ul>
      |     <li>init_pos: Initial wheel center position (global x, y and z
      | coordinate)</li>
      |     <li>init_angle: Initial wheel center orientation (global, Bryant angles, rotation
      |     seq. ZXY). Angle input order [X Y Z]. </li>
      | </ul>
      | <hr WIDTH="100%">
      | <br><font size=+1>General notes:</font>
      | <ul>
      | <li>
      | All calculations are made using SI-units (m, rad, N, kg, s)<br>&nbsp;</li>
      | 
      | </ul>
      | ©1996-2011 TNO Automotive, The Netherlands
      | </body>
      | </html>

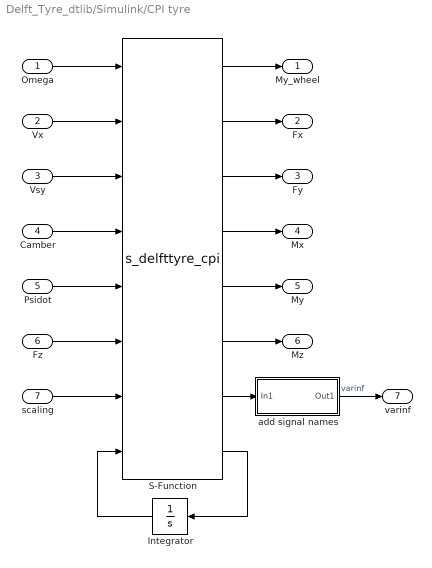
== system Delft_Tyre_dtlib/Simulink/CPI tyre ==
  Omega : Inport  OutDataType=fixdt(1,16,0)  OutScaling=[]
  Vx : Inport  Port=2  OutDataType=fixdt(1,16,0)  OutScaling=[]
  Vsy : Inport  Port=3  OutDataType=fixdt(1,16,0)  OutScaling=[]
  Camber : Inport  Port=4  OutDataType=fixdt(1,16,0)  OutScaling=[]
  Psidot : Inport  Port=5  OutDataType=fixdt(1,16,0)  OutScaling=[]
  Fz : Inport  Port=6  OutDataType=fixdt(1,16,0)  OutScaling=[]
  scaling : Inport  Port=7  OutDataType=fixdt(1,16,0)  OutScaling=[]
  Integrator : Integrator  Orientation=left  InitialCondition=zeros(1,17)
  S-Function : S-Function  FunctionName=s_delfttyre_cpi  Parameters=iswtch idtyre tpfname
  add signal names : Subsystem
  My_wheel : Outport  OutDataType=fixdt(1,16,0)  OutScaling=[]
  Fx : Outport  Port=2  OutDataType=fixdt(1,16,0)  OutScaling=[]
  Fy : Outport  Port=3  OutDataType=fixdt(1,16,0)  OutScaling=[]
  Mx : Outport  Port=4  OutDataType=fixdt(1,16,0)  OutScaling=[]
  My : Outport  Port=5  OutDataType=fixdt(1,16,0)  OutScaling=[]
  Mz : Outport  Port=6  OutDataType=fixdt(1,16,0)  OutScaling=[]
  varinf : Outport  Port=7  OutDataType=fixdt(1,16,0)  OutScaling=[]
  wires:
  add signal names/1(Out1) -> varinf/1  "varinf"
  S-Function/7 -> add signal names/1(In1)
  scaling/1 -> S-Function/7
  Integrator/1 -> S-Function/8
  S-Function/8 -> Integrator/1
  Omega/1 -> S-Function/1
  Vx/1 -> S-Function/2
  Vsy/1 -> S-Function/3
  Camber/1 -> S-Function/4
  Psidot/1 -> S-Function/5
  Fz/1 -> S-Function/6
  S-Function/1 -> My_wheel/1
  S-Function/2 -> Fx/1
  S-Function/3 -> Fy/1
  S-Function/4 -> Mx/1
  S-Function/5 -> My/1
  S-Function/6 -> Mz/1

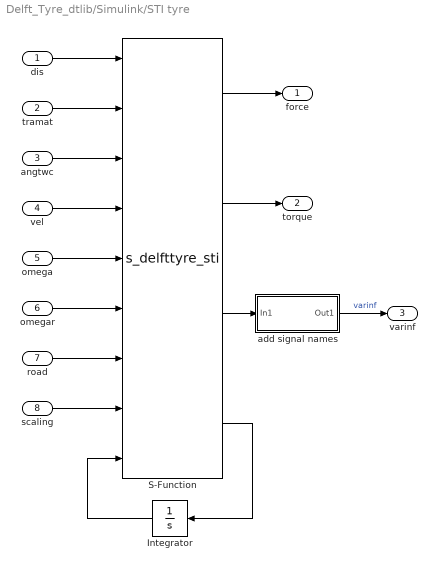
== system Delft_Tyre_dtlib/Simulink/STI tyre ==
  dis : Inport  OutDataType=fixdt(1,16,0)  OutScaling=[]
  tramat : Inport  Port=2  OutDataType=fixdt(1,16,0)  OutScaling=[]
  angtwc : Inport  Port=3  OutDataType=fixdt(1,16,0)  OutScaling=[]
  vel : Inport  Port=4  OutDataType=fixdt(1,16,0)  OutScaling=[]
  omega : Inport  Port=5  OutDataType=fixdt(1,16,0)  OutScaling=[]
  omegar : Inport  Port=6  OutDataType=fixdt(1,16,0)  OutScaling=[]
  road : Inport  Port=7  OutDataType=fixdt(1,16,0)  OutScaling=[]
  scaling : Inport  Port=8  OutDataType=fixdt(1,16,0)  OutScaling=[]
  Integrator : Integrator  Orientation=left  InitialCondition=zeros(1,40)
  S-Function : S-Function  FunctionName=s_delfttyre_sti  Parameters=iswtch idtyre idroad tpfname_dummy rdfname typarr
  add signal names : Subsystem
  force : Outport  OutDataType=fixdt(1,16,0)  OutScaling=[]
  torque : Outport  Port=2  OutDataType=fixdt(1,16,0)  OutScaling=[]
  varinf : Outport  Port=3  OutDataType=fixdt(1,16,0)  OutScaling=[]
  wires:
  tramat/1 -> S-Function/2
  angtwc/1 -> S-Function/3
  vel/1 -> S-Function/4
  omega/1 -> S-Function/5
  omegar/1 -> S-Function/6
  road/1 -> S-Function/7
  dis/1 -> S-Function/1
  S-Function/2 -> torque/1
  S-Function/1 -> force/1
  S-Function/4 -> Integrator/1
  Integrator/1 -> S-Function/9
  scaling/1 -> S-Function/8
  S-Function/3 -> add signal names/1(In1)
  add signal names/1(Out1) -> varinf/1  "varinf"

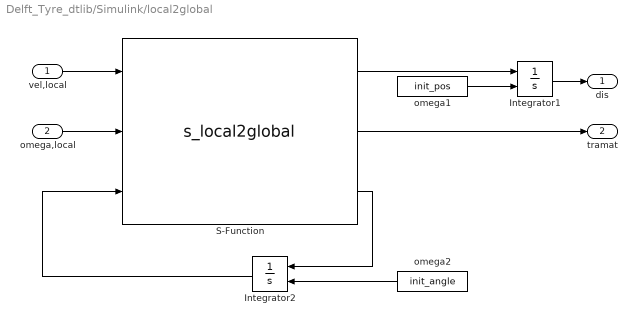
== system Delft_Tyre_dtlib/Simulink/local2global ==
  vel,local : Inport  OutDataType=fixdt(1,16,0)  OutScaling=[]
  omega,local : Inport  Port=2  OutDataType=fixdt(1,16,0)  OutScaling=[]
  Integrator1 : Integrator  InitialConditionSource=external
  Integrator2 : Integrator  Orientation=left  InitialConditionSource=external
  S-Function : S-Function  FunctionName=s_local2global
  omega1 : Constant  Value=init_pos  OutDataType=fixdt(1,16,0)  ConRadixGroup=Use specified scaling  OutScaling=[]  SampleTime=inf  FramePeriod=inf
  omega2 : Constant  Orientation=left  Value=init_angle  OutDataType=fixdt(1,16,0)  ConRadixGroup=Use specified scaling  OutScaling=[]  SampleTime=inf  FramePeriod=inf
  dis : Outport  OutDataType=fixdt(1,16,0)  OutScaling=[]
  tramat : Outport  Port=2  OutDataType=fixdt(1,16,0)  OutScaling=[]
  wires:
  vel,local/1 -> S-Function/1
  omega,local/1 -> S-Function/2
  Integrator1/1 -> dis/1
  omega1/1 -> Integrator1/2
  omega2/1 -> Integrator2/2
  Integrator2/1 -> S-Function/3
  S-Function/2 -> tramat/1
  S-Function/1 -> Integrator1/1
  S-Function/3 -> Integrator2/1

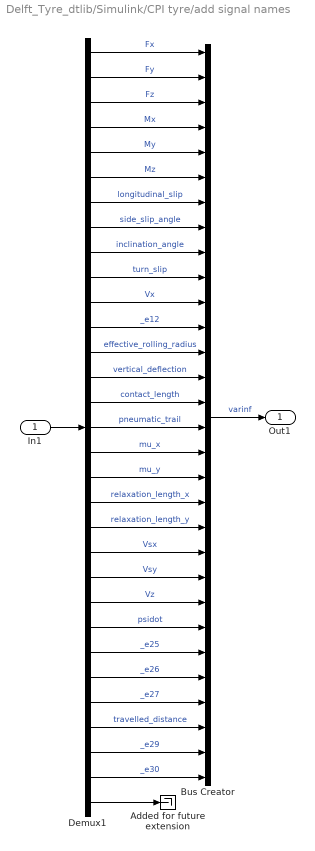
== system Delft_Tyre_dtlib/Simulink/CPI tyre/add signal names ==
  In1 : Inport  OutDataType=fixdt(1,16,0)  OutScaling=[]
  Added for future extension : Terminator
  Bus Creator : BusCreator  Inputs=30
  Demux1 : Demux  Outputs=[ones(1,30) -1]
  Out1 : Outport  OutDataType=fixdt(1,16,0)  OutScaling=[]
  wires:
  In1/1 -> Demux1/1
  Demux1/1 -> Bus Creator/1  "Fx"
  Demux1/2 -> Bus Creator/2  "Fy"
  Demux1/3 -> Bus Creator/3  "Fz"
  Demux1/4 -> Bus Creator/4  "Mx"
  Demux1/5 -> Bus Creator/5  "My"
  Demux1/6 -> Bus Creator/6  "Mz"
  Demux1/7 -> Bus Creator/7  "longitudinal_slip"
  Demux1/8 -> Bus Creator/8  "side_slip_angle"
  Demux1/9 -> Bus Creator/9  "inclination_angle"
  Demux1/10 -> Bus Creator/10  "turn_slip"
  Demux1/11 -> Bus Creator/11  "Vx"
  Demux1/12 -> Bus Creator/12  "_e12"
  Demux1/13 -> Bus Creator/13  "effective_rolling_radius"
  Demux1/14 -> Bus Creator/14  "vertical_deflection"
  Demux1/15 -> Bus Creator/15  "contact_length"
  Demux1/16 -> Bus Creator/16  "pneumatic_trail"
  Demux1/17 -> Bus Creator/17  "mu_x"
  Demux1/18 -> Bus Creator/18  "mu_y"
  Demux1/19 -> Bus Creator/19  "relaxation_length_x"
  Demux1/20 -> Bus Creator/20  "relaxation_length_y"
  Demux1/21 -> Bus Creator/21  "Vsx"
  Demux1/22 -> Bus Creator/22  "Vsy"
  Demux1/23 -> Bus Creator/23  "Vz"
  Demux1/24 -> Bus Creator/24  "psidot"
  Demux1/25 -> Bus Creator/25  "_e25"
  Demux1/26 -> Bus Creator/26  "_e26"
  Demux1/27 -> Bus Creator/27  "_e27"
  Demux1/28 -> Bus Creator/28  "travelled_distance"
  Demux1/29 -> Bus Creator/29  "_e29"
  Demux1/30 -> Bus Creator/30  "_e30"
  Bus Creator/1 -> Out1/1  "varinf"
  Demux1/31 -> Added for future extension/1

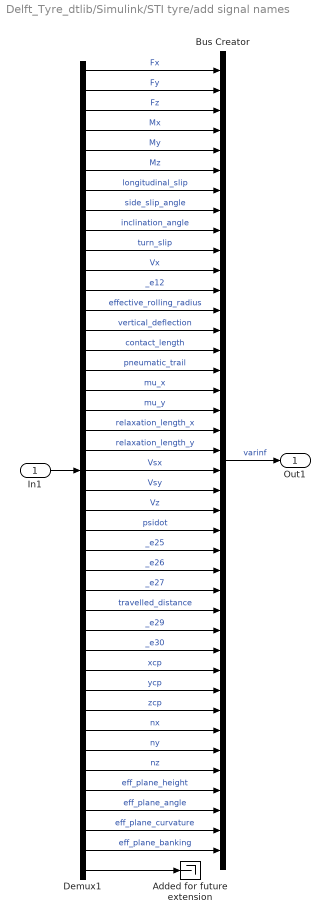
== system Delft_Tyre_dtlib/Simulink/STI tyre/add signal names ==
  In1 : Inport  OutDataType=fixdt(1,16,0)  OutScaling=[]
  Added for future extension : Terminator
  Bus Creator : BusCreator  Inputs=40
  Demux1 : Demux  Outputs=[ones(1,40) -1]
  Out1 : Outport  OutDataType=fixdt(1,16,0)  OutScaling=[]
  wires:
  In1/1 -> Demux1/1
  Bus Creator/1 -> Out1/1  "varinf"
  Demux1/1 -> Bus Creator/1  "Fx"
  Demux1/2 -> Bus Creator/2  "Fy"
  Demux1/3 -> Bus Creator/3  "Fz"
  Demux1/4 -> Bus Creator/4  "Mx"
  Demux1/5 -> Bus Creator/5  "My"
  Demux1/6 -> Bus Creator/6  "Mz"
  Demux1/7 -> Bus Creator/7  "longitudinal_slip"
  Demux1/8 -> Bus Creator/8  "side_slip_angle"
  Demux1/9 -> Bus Creator/9  "inclination_angle"
  Demux1/10 -> Bus Creator/10  "turn_slip"
  Demux1/11 -> Bus Creator/11  "Vx"
  Demux1/12 -> Bus Creator/12  "_e12"
  Demux1/13 -> Bus Creator/13  "effective_rolling_radius"
  Demux1/14 -> Bus Creator/14  "vertical_deflection"
  Demux1/15 -> Bus Creator/15  "contact_length"
  Demux1/16 -> Bus Creator/16  "pneumatic_trail"
  Demux1/17 -> Bus Creator/17  "mu_x"
  Demux1/18 -> Bus Creator/18  "mu_y"
  Demux1/19 -> Bus Creator/19  "relaxation_length_x"
  Demux1/20 -> Bus Creator/20  "relaxation_length_y"
  Demux1/21 -> Bus Creator/21  "Vsx"
  Demux1/22 -> Bus Creator/22  "Vsy"
  Demux1/23 -> Bus Creator/23  "Vz"
  Demux1/24 -> Bus Creator/24  "psidot"
  Demux1/25 -> Bus Creator/25  "_e25"
  Demux1/26 -> Bus Creator/26  "_e26"
  Demux1/27 -> Bus Creator/27  "_e27"
  Demux1/28 -> Bus Creator/28  "travelled_distance"
  Demux1/29 -> Bus Creator/29  "_e29"
  Demux1/30 -> Bus Creator/30  "_e30"
  Demux1/31 -> Bus Creator/31  "xcp"
  Demux1/32 -> Bus Creator/32  "ycp"
  Demux1/33 -> Bus Creator/33  "zcp"
  Demux1/34 -> Bus Creator/34  "nx"
  Demux1/35 -> Bus Creator/35  "ny"
  Demux1/36 -> Bus Creator/36  "nz"
  Demux1/37 -> Bus Creator/37  "eff_plane_height"
  Demux1/38 -> Bus Creator/38  "eff_plane_angle"
  Demux1/39 -> Bus Creator/39  "eff_plane_curvature"
  Demux1/40 -> Bus Creator/40  "eff_plane_banking"
  Demux1/41 -> Added for future extension/1
